simulink model "Exercitiul1"  (R2016a)
settings: Solver=VariableStepDiscrete  StartTime=0.0  StopTime=50  RelTol=1e-3
undefined symbols (not defined in the file): m, n
settings Model: Creator=Cristina  LastModifiedBy=Cristina

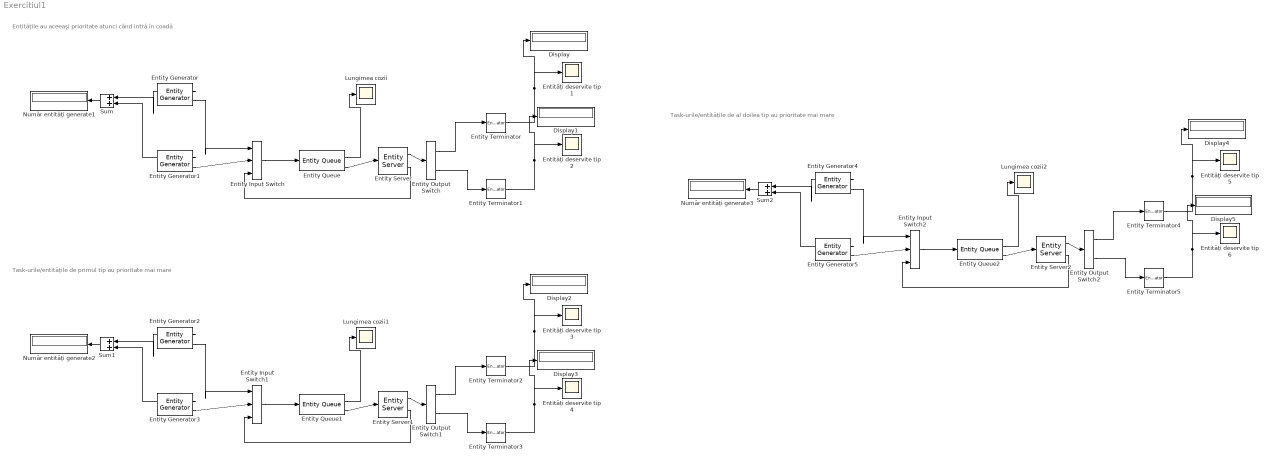
== system Exercitiul1 ==
  note: Entitățile au aceeași prioritate atunci când intră în coadă
  note: Task-urile/entitățile de primul tip au prioritate mai mare
  note: Task-urile/entitățile de al doilea tip au prioritate mai mare
  Display{,1..5} (6 alike) : Display
  Entity Input Switch : EntityInputSwitch  InputPortMessageModes=m,m,m  OutputPortMessageModes=m  NumberInputPorts=3
      settings: InputPortMap=u1,u2,u3
  Entity Input Switch1 : EntityInputSwitch  InputPortMessageModes=m,m,m  OutputPortMessageModes=m  NumberInputPorts=3
      settings: InputPortMap=u1,u2,u3
  Entity Input Switch2 : EntityInputSwitch  InputPortMessageModes=m,m,m  OutputPortMessageModes=m  NumberInputPorts=3
      settings: InputPortMap=u1,u2,u3
  Entity Output Switch : EntityOutputSwitch  InputPortMessageModes=m  OutputPortMessageModes=m,m  SwitchingCriterion=From attribute  SwitchAttributeName=Type
  Entity Output Switch1 : EntityOutputSwitch  InputPortMessageModes=m  OutputPortMessageModes=m,m  SwitchingCriterion=From attribute  SwitchAttributeName=Type
  Entity Output Switch2 : EntityOutputSwitch  InputPortMessageModes=m  OutputPortMessageModes=m,m  SwitchingCriterion=From attribute  SwitchAttributeName=Type
  Entity Generator : EntityGenerator  OutputPortMessageModes=n,m  Period=2  AttributeName=ServiceTime|Type|Priority  AttributeInitialValue=1|1|1  NumberEntitiesDeparted=on  EntityType=Structured  EntityTypeName=Entity
      settings: OutputPortMap=o0,o3
  Entity Generator1 : EntityGenerator  OutputPortMessageModes=n,m  Period=5  AttributeName=ServiceTime|Type|Priority  AttributeInitialValue=2.5|2|1  NumberEntitiesDeparted=on  EntityType=Structured  EntityTypeName=Entity
      settings: OutputPortMap=o0,o3
  Entity Generator2 : EntityGenerator  OutputPortMessageModes=n,m  Period=2  AttributeName=ServiceTime|Type|Priority  AttributeInitialValue=1|1|1  NumberEntitiesDeparted=on  EntityType=Structured  EntityTypeName=Entity
      settings: OutputPortMap=o0,o3
  Entity Generator3 : EntityGenerator  OutputPortMessageModes=n,m  Period=5  AttributeName=ServiceTime|Type|Priority  AttributeInitialValue=2.5|2|2  NumberEntitiesDeparted=on  EntityType=Structured  EntityTypeName=Entity
      settings: OutputPortMap=o0,o3
  Entity Generator4 : EntityGenerator  OutputPortMessageModes=n,m  Period=2  AttributeName=ServiceTime|Type|Priority  AttributeInitialValue=1|1|2  NumberEntitiesDeparted=on  EntityType=Structured  EntityTypeName=Entity
      settings: OutputPortMap=o0,o3
  Entity Generator5 : EntityGenerator  OutputPortMessageModes=n,m  Period=5  AttributeName=ServiceTime|Type|Priority  AttributeInitialValue=2.5|2|1  NumberEntitiesDeparted=on  EntityType=Structured  EntityTypeName=Entity
      settings: OutputPortMap=o0,o3
  Entity Queue : EntityQueue  InputPortMessageModes=m  OutputPortMessageModes=n,m  QueueType=Priority  PrioritySource=Priority  AverageQueueLength=on
      settings: OutputPortMap=o3,o5
  Entity Queue1 : EntityQueue  InputPortMessageModes=m  OutputPortMessageModes=n,m  QueueType=Priority  PrioritySource=Priority  AverageQueueLength=on
      settings: OutputPortMap=o3,o5
  Entity Queue2 : EntityQueue  InputPortMessageModes=m  OutputPortMessageModes=n,m  QueueType=Priority  PrioritySource=Priority  AverageQueueLength=on
      settings: OutputPortMap=o3,o5
  Entity Server : EntityServer  InputPortMessageModes=m  OutputPortMessageModes=m,m  Capacity=1  ServiceTimeSource=Attribute  PermitPreemptionBasedOnAttribute=on  SortingAttributeName=Priority  SortingDirection=Descending  WriteResidualTimeToAttribute=on  ResidualTimeAttributeName=ServiceTime
      settings: OutputPortMap=o9,o10
  Entity Server1 : EntityServer  InputPortMessageModes=m  OutputPortMessageModes=m,m  Capacity=1  ServiceTimeSource=Attribute  PermitPreemptionBasedOnAttribute=on  SortingAttributeName=Priority  SortingDirection=Descending  WriteResidualTimeToAttribute=on  ResidualTimeAttributeName=ServiceTime
      settings: OutputPortMap=o9,o10
  Entity Server2 : EntityServer  InputPortMessageModes=m  OutputPortMessageModes=m,m  Capacity=1  ServiceTimeSource=Attribute  PermitPreemptionBasedOnAttribute=on  SortingAttributeName=Priority  SortingDirection=Descending  WriteResidualTimeToAttribute=on  ResidualTimeAttributeName=ServiceTime
      settings: OutputPortMap=o9,o10
  Entity Terminator{,1..5} (6 alike) : EntityTerminator  InputPortMessageModes=m  NumberEntitiesArrived=on
      settings: OutputPortMap=o0
  Entități deservite tip {1..6} (6 alike) : Scope
  Lungimea cozii : Scope
  Lungimea cozii1 : Scope
  Lungimea cozii2 : Scope
  Număr entități generate1 : Display
  Număr entități generate2 : Display
  Număr entități generate3 : Display
  Sum : Sum  Inputs=|++
  Sum1 : Sum  Inputs=|++
  Sum2 : Sum  Inputs=|++
  wires:
  Entity Input Switch/1 -> Entity Queue/1
  Entity Generator1/2 -> Entity Input Switch/2
  Entity Generator/2 -> Entity Input Switch/1
  Entity Server/2 -> Entity Input Switch/3
  Entity Generator/1 -> Sum/1
  Entity Generator1/1 -> Sum/2
  Entity Server/1 -> Entity Output Switch/1
  Entity Queue/2 -> Entity Server/1
  Entity Queue/1 -> Lungimea cozii/1
  Entity Output Switch/1 -> Entity Terminator/1
  Entity Output Switch/2 -> Entity Terminator1/1
  Entity Terminator/1 -> Display/1, Entități deservite tip 1/1
  Entity Terminator1/1 -> Display1/1, Entități deservite tip 2/1
  Sum/1 -> Număr entități generate1/1
  Entity Input Switch1/1 -> Entity Queue1/1
  Entity Generator3/2 -> Entity Input Switch1/2
  Entity Generator2/2 -> Entity Input Switch1/1
  Entity Server1/2 -> Entity Input Switch1/3
  Entity Generator2/1 -> Sum1/1
  Entity Generator3/1 -> Sum1/2
  Entity Server1/1 -> Entity Output Switch1/1
  Entity Queue1/2 -> Entity Server1/1
  Entity Queue1/1 -> Lungimea cozii1/1
  Entity Output Switch1/1 -> Entity Terminator2/1
  Entity Output Switch1/2 -> Entity Terminator3/1
  Entity Terminator2/1 -> Entități deservite tip 3/1, Display2/1
  Entity Terminator3/1 -> Entități deservite tip 4/1, Display3/1
  Sum1/1 -> Număr entități generate2/1
  Entity Input Switch2/1 -> Entity Queue2/1
  Entity Generator5/2 -> Entity Input Switch2/2
  Entity Generator4/2 -> Entity Input Switch2/1
  Entity Server2/2 -> Entity Input Switch2/3
  Entity Generator4/1 -> Sum2/1
  Entity Generator5/1 -> Sum2/2
  Entity Server2/1 -> Entity Output Switch2/1
  Entity Queue2/2 -> Entity Server2/1
  Entity Queue2/1 -> Lungimea cozii2/1
  Entity Output Switch2/1 -> Entity Terminator4/1
  Entity Output Switch2/2 -> Entity Terminator5/1
  Entity Terminator4/1 -> Display4/1, Entități deservite tip 5/1
  Entity Terminator5/1 -> Display5/1, Entități deservite tip 6/1
  Sum2/1 -> Număr entități generate3/1
